simulink model "PAM"  (R2020b)
settings: Solver=VariableStepAuto  StartTime=0.0  StopTime=0.05  RelTol=1e-3
libraries: dsparch4 x2, dspsigops x1
settings Model: Creator=EASY LIFE  LastModifiedBy=LENOVO

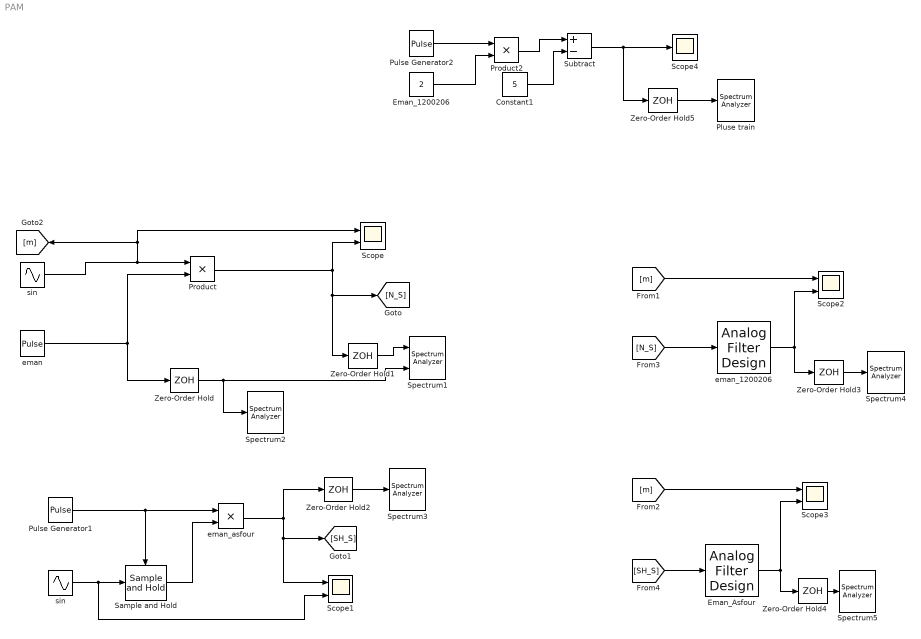
== system PAM ==
  " sin" : Sin  Amplitude=5  Frequency=1000*2*pi  SampleTime=0
  Constant1 : Constant  Value=5
  Eman_1200206 : Constant  Value=2
  Eman_Asfour : dsparch4/Analog Filter Design  method=Butterworth  filttype=Lowpass  N=8  Wlo=2*pi*1000*1.1  Whi=80  Rp=2  Rs=40
  "Pluse train " : SpectrumAnalyzer
  Product : Product
  Product2 : Product
  Pulse Generator1 : DiscretePulseGenerator  PulseType=Time based  Period=1/5000  PulseWidth=50
  Pulse Generator2 : DiscretePulseGenerator  PulseType=Time based  Amplitude=5  Period=0.001  PulseWidth=90
  Sample and Hold : dspsigops/Sample and Hold  trig=Rising edge  initCond=0  latchinput=off
  Scope{,1..3} (4 alike) : Scope  NumInputPorts=2
  Scope4 : Scope
  Spectrum1 : SpectrumAnalyzer  NumInputPorts=2
  Spectrum{2..5} (4 alike) : SpectrumAnalyzer
  Subtract : Sum  Inputs=+-
  Zero-Order Hold : ZeroOrderHold  SampleTime=1/50000
  Zero-Order Hold1 : ZeroOrderHold  SampleTime=1/50000
  Zero-Order Hold2 : ZeroOrderHold  SampleTime=1/50000
  Zero-Order Hold3 : ZeroOrderHold  SampleTime=1/5000
  Zero-Order Hold4 : ZeroOrderHold  SampleTime=-1
  Zero-Order Hold5 : ZeroOrderHold  SampleTime=1/100000
  eman : DiscretePulseGenerator  PulseType=Time based  Period=1/5000  PulseWidth=50
  eman_1200206 : dsparch4/Analog Filter Design  method=Butterworth  filttype=Lowpass  N=8  Wlo=2*pi*1000*1.1  Whi=80  Rp=2  Rs=40
  eman_asfour : Product
  "sin " : Sin  Amplitude=5  Frequency=3000*2*pi  SampleTime=0
  wires:
  eman/1 -> Zero-Order Hold/1, Product/2
  Zero-Order Hold/1 -> Spectrum2/1, Spectrum1/2
  Product/1 -> Zero-Order Hold1/1, [N_S], Scope/2
  Zero-Order Hold1/1 -> Spectrum1/1
  "sin "/1 -> Product/1, [m], Scope/1
  Zero-Order Hold2/1 -> Spectrum3/1
  eman_asfour/1 -> Scope1/1, [SH_S], Zero-Order Hold2/1
  Pulse Generator1/1 -> Sample and Hold/Trigger, eman_asfour/1
  " sin"/1 -> Scope1/2, Sample and Hold/1
  Sample and Hold/1 -> eman_asfour/2
  [N_S] -> eman_1200206/1
  [m] -> Scope2/1
  eman_1200206/1 -> Zero-Order Hold3/1, Scope2/2
  Zero-Order Hold3/1 -> Spectrum4/1
  [m] -> Scope3/1
  [SH_S] -> Eman_Asfour/1
  Eman_Asfour/1 -> Zero-Order Hold4/1, Scope3/2
  Zero-Order Hold4/1 -> Spectrum5/1
  Eman_1200206/1 -> Product2/2
  Zero-Order Hold5/1 -> "Pluse train "/1
  Constant1/1 -> Subtract/2
  Pulse Generator2/1 -> Product2/1
  Subtract/1 -> Zero-Order Hold5/1, Scope4/1
  Product2/1 -> Subtract/1
